simulink model "MATLAB_accumulator_tester"  (R2022a)
settings: Solver=FixedStepDiscrete  StartTime=0.0  StopTime=inf  FixedStep=Ts  MaxStep=0.001  RelTol=1e-3
PreLoadFcn:
  | load 'MATLAB_accumulator_tester_wrksp.mat'
model workspace (MAT data in the model file):
  MAX_V = Simulink.Parameter
  MAX_V.Value = 31
  MAX_V.DataType = 'single'
  MAX_V.Complexity = 'real'
  MAX_V.Dimensions = [1 1]
  MIN_ACCUM_VOLTAGE = Simulink.Parameter
  MIN_ACCUM_VOLTAGE.Value = 10
  MIN_ACCUM_VOLTAGE.DataType = 'single'
  MIN_ACCUM_VOLTAGE.Complexity = 'real'
  MIN_ACCUM_VOLTAGE.Dimensions = [1 1]
  TARGET_ACCUM_CURRENT = Simulink.Parameter
  TARGET_ACCUM_CURRENT.Value = 6
  TARGET_ACCUM_CURRENT.DataType = 'single'
  TARGET_ACCUM_CURRENT.Complexity = 'real'
  TARGET_ACCUM_CURRENT.Dimensions = [1 1]
values from neighbouring files (symbols this model uses):
  Ts = 0.01    [MATLAB_accumulator_tester_wrksp.mat]
undefined symbols (not defined in the file or in its folder): CR, d, f, LF
libraries: simulink x5, slrealtimeutilitieslib x3, instrumentlib x2, dspstat3 x2, commcrc2 x1
settings Model: SimulationMode=accelerator  Creator=DeveloperY  LastModifiedBy=DeveloperY
settings SolverCC: AllowMultiTaskInputOutput=on  ConcurrentTasks=on  AutoInsertRateTranBlk=on
settings DebuggingCC: ParameterPrecisionLossMsg=none
settings HardwareCC: ProdBitPerLong=64  ProdHWDeviceType=Intel->x86-64 (Linux 64)
settings RTWCC: Description=Simulink Desktop Real-Time  SystemTargetFile=sldrt.tlc  TemplateMakefile=sldrt.tmf  RTWCompilerOptimization=on
settings CodeAppCC: MaxIdLength=95
settings SimulinkDesktopRealTimeCC: TargetLibSuffix=_sldrt.a  TargetPreCompLibLocation=C:\Program Files\MATLAB\R2022a\toolbox\sldrt\lib\win64  RebuildAll=on

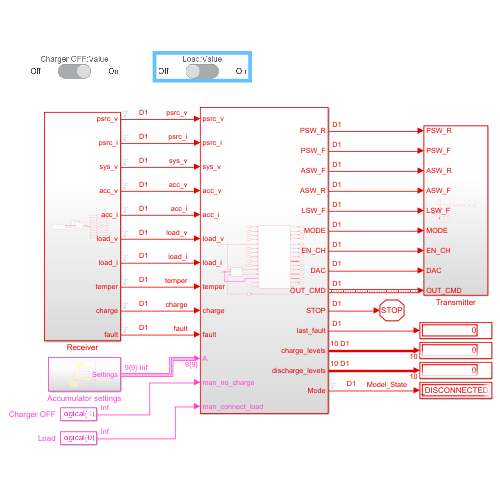
[thumbnail: Simulink's stored preview of the top-level diagram]
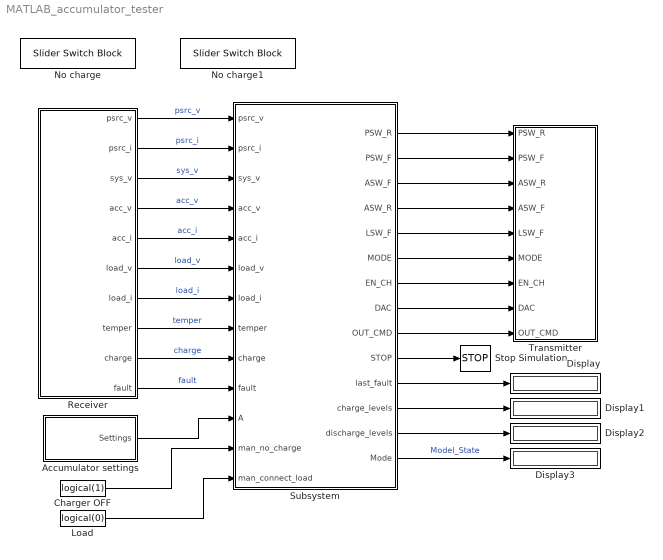
== system MATLAB_accumulator_tester ==
  Accumulator settings : Subsystem
  Charger OFF : Constant  Value=logical(1)  OutDataTypeStr=boolean
  Display{,1..3} (4 alike) : Display
  Load : Constant  Value=logical(0)  OutDataTypeStr=boolean
  No charge : SliderSwitchBlock
      settings: Values={{'Off', 'On'}, [0 1]}
  No charge1 : SliderSwitchBlock
      settings: Values={{'Off', 'On'}, [0 1]}
  Receiver : Subsystem
  Stop Simulation : Stop
  Subsystem : Subsystem
  Transmitter : Subsystem
  wires:
  Receiver/1(psrc_v) -> Subsystem/1(psrc_v)  "psrc_v"
  Receiver/2(psrc_i) -> Subsystem/2(psrc_i)  "psrc_i"
  Receiver/3(sys_v) -> Subsystem/3(sys_v)  "sys_v"
  Receiver/4(acc_v) -> Subsystem/4(acc_v)  "acc_v"
  Receiver/5(acc_i) -> Subsystem/5(acc_i)  "acc_i"
  Receiver/6(load_v) -> Subsystem/6(load_v)  "load_v"
  Receiver/7(load_i) -> Subsystem/7(load_i)  "load_i"
  Receiver/8(temper) -> Subsystem/8(temper)  "temper"
  Subsystem/1(PSW_R) -> Transmitter/1(PSW_R)
  Subsystem/2(PSW_F) -> Transmitter/2(PSW_F)
  Subsystem/3(ASW_F) -> Transmitter/3(ASW_R)
  Subsystem/4(ASW_R) -> Transmitter/4(ASW_F)
  Subsystem/5(LSW_F) -> Transmitter/5(LSW_F)
  Subsystem/6(MODE) -> Transmitter/6(MODE)
  Subsystem/7(EN_CH) -> Transmitter/7(EN_CH)
  Subsystem/8(DAC) -> Transmitter/8(DAC)
  Receiver/10(fault) -> Subsystem/10(fault)  "fault"
  Subsystem/10(" STOP") -> Stop Simulation/1
  Subsystem/11(last_fault) -> Display/1
  Accumulator settings/1(Settings) -> Subsystem/11(A)
  Receiver/9(charge) -> Subsystem/9(charge)  "charge"
  Subsystem/12(charge_levels) -> Display1/1
  Subsystem/13(discharge_levels) -> Display2/1
  Subsystem/14(Mode) -> Display3/1  "Model_State"
  Subsystem/9(OUT_CMD) -> Transmitter/9(OUT_CMD)
  Charger OFF/1 -> Subsystem/12(man_no_charge)
  Load/1 -> Subsystem/13(man_connect_load)

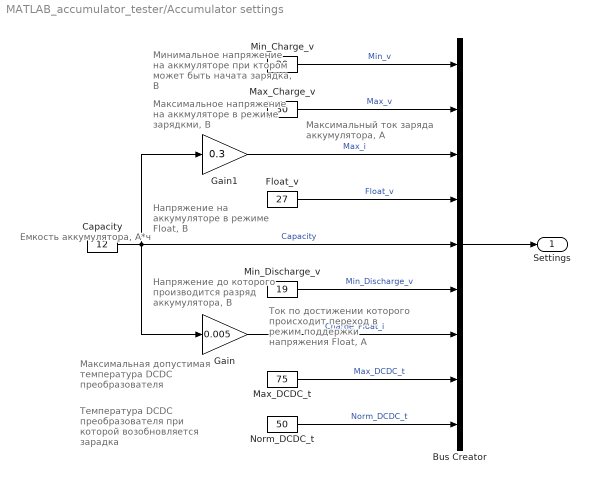
== system MATLAB_accumulator_tester/Accumulator settings ==
  note: Ток по достижении которого происходит переход в режим поддержки напряжения Float, А
  note: Максимальная допустимая температура DCDC преобразователя
  note: Температура DCDC преобразователя при которой возобновляется зарадка
  note: Напряжение до которого производится разряд аккумулятора, В
  note: Емкость аккумулятора, А*ч
  note: Напряжение на аккумуляторе в режиме Float, В
  note: Максимальное напряжение на аккмуляторе в режиме зарядкми, В
  note: Максимальный ток заряда аккумулятора, А
  note: Минимальное напряжение на аккмуляторе при ктором может быть начата зарядка, В
  Bus Creator : BusCreator  Inputs=9  OutDataTypeStr=Bus: Accum_params
  Capacity : Constant  Value=12  OutDataTypeStr=single
  Float_v : Constant  Value=27  OutDataTypeStr=single
  Gain : Gain  Gain=0.005
  Gain1 : Gain  Gain=0.3
  Max_Charge_v : Constant  Value=30  OutDataTypeStr=single
  Max_DCDC_t : Constant  Value=75  OutDataTypeStr=single
  Min_Charge_v : Constant  Value=20  OutDataTypeStr=single
  Min_Discharge_v : Constant  Value=19  OutDataTypeStr=single
  Norm_DCDC_t : Constant  Value=50  OutDataTypeStr=single
  Settings : Outport
  wires:
  Bus Creator/1 -> Settings/1
  Gain1/1 -> Bus Creator/3  "Max_i"
  Capacity/1 -> Gain/1, Gain1/1, Bus Creator/5  "Capacity"
  Max_Charge_v/1 -> Bus Creator/2  "Max_v"
  Float_v/1 -> Bus Creator/4  "Float_v"
  Min_Charge_v/1 -> Bus Creator/1  "Min_v"
  Min_Discharge_v/1 -> Bus Creator/6  "Min_Discharge_v"
  Gain/1 -> Bus Creator/7  "Charge_Float_i"
  Max_DCDC_t/1 -> Bus Creator/8  "Max_DCDC_t"
  Norm_DCDC_t/1 -> Bus Creator/9  "Norm_DCDC_t"

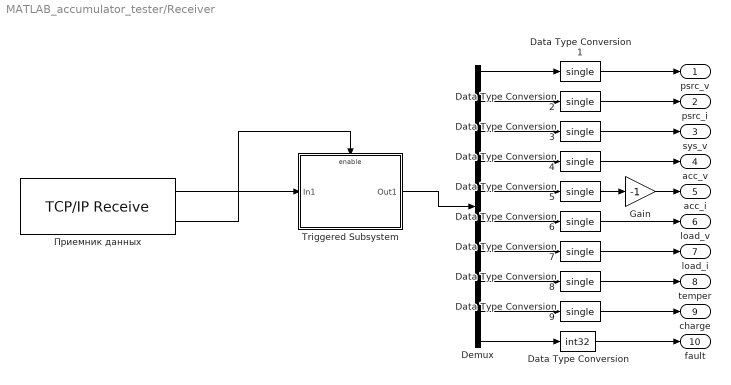
== system MATLAB_accumulator_tester/Receiver ==
  Data Type Conversion : DataTypeConversion  OutDataTypeStr=int32  SaturateOnIntegerOverflow=off  RndMeth=Floor
  Data Type Conversion{1..9} (9 alike) : DataTypeConversion  OutDataTypeStr=single  SaturateOnIntegerOverflow=off  RndMeth=Floor
  Demux : Demux  Outputs=10
  Gain : Gain  Gain=-1
  Triggered Subsystem : Subsystem  TreatAsAtomicUnit=on
  Приемник данных : instrumentlib/TCP//IP Receive  Host=192.168.3.1  Port=3333  DataSize=[10]  DataType=ASCII  ASCIIFormatting=%f,%f,%f,%f,%f,%f,%f,%f,%e,%d  Terminator=CR/LF  CustomTerminator=10  ByteOrder=big-endian  EnableBlockingMode=off  Timeout=10  SampleTime=-1  SimulateUsing=Interpreted execution
  psrc_v : Outport
  psrc_i : Outport  Port=2
  sys_v : Outport  Port=3
  acc_v : Outport  Port=4
  acc_i : Outport  Port=5
  load_v : Outport  Port=6
  load_i : Outport  Port=7
  temper : Outport  Port=8
  charge : Outport  Port=9
  fault : Outport  Port=10
  wires:
  Demux/4 -> Data Type Conversion4/1
  Demux/5 -> Data Type Conversion5/1
  Приемник данных/1 -> Triggered Subsystem/1(In1)
  Приемник данных/2 -> Triggered Subsystem/Enable
  Demux/6 -> Data Type Conversion6/1
  Demux/1 -> Data Type Conversion1/1
  Triggered Subsystem/1(Out1) -> Demux/1
  Demux/2 -> Data Type Conversion2/1
  Demux/8 -> Data Type Conversion8/1
  Demux/7 -> Data Type Conversion7/1
  Demux/3 -> Data Type Conversion3/1
  Demux/10 -> Data Type Conversion/1
  Data Type Conversion/1 -> fault/1
  Data Type Conversion1/1 -> psrc_v/1
  Data Type Conversion2/1 -> psrc_i/1
  Data Type Conversion3/1 -> sys_v/1
  Data Type Conversion4/1 -> acc_v/1
  Data Type Conversion5/1 -> Gain/1
  Data Type Conversion6/1 -> load_v/1
  Data Type Conversion7/1 -> load_i/1
  Data Type Conversion8/1 -> temper/1
  Gain/1 -> acc_i/1
  Demux/9 -> Data Type Conversion9/1
  Data Type Conversion9/1 -> charge/1

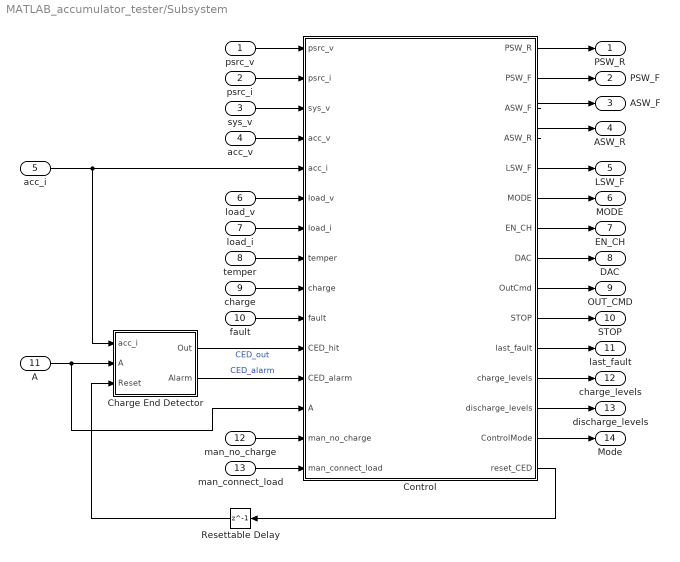
== system MATLAB_accumulator_tester/Subsystem ==
  psrc_v : Inport
  psrc_i : Inport  Port=2
  sys_v : Inport  Port=3
  acc_v : Inport  Port=4
  acc_i : Inport  Port=5
  load_v : Inport  Port=6
  load_i : Inport  Port=7
  temper : Inport  Port=8
  charge : Inport  Port=9
  fault : Inport  Port=10
  A : Inport  Port=11
  man_no_charge : Inport  Port=12
  man_connect_load : Inport  Port=13
  Charge End Detector : Subsystem
  Control : Stateflow chart  TreatAsAtomicUnit=on
  Resettable Delay : Delay  DelayLength=1
  PSW_R : Outport
  PSW_F : Outport  Port=2
  ASW_F : Outport  Port=3
  ASW_R : Outport  Port=4
  LSW_F : Outport  Port=5
  MODE : Outport  Port=6
  EN_CH : Outport  Port=7
  DAC : Outport  Port=8
  OUT_CMD : Outport  Port=9
  " STOP" : Outport  Port=10
  last_fault : Outport  Port=11
  charge_levels : Outport  Port=12
  discharge_levels : Outport  Port=13
  Mode : Outport  Port=14
  wires:
  psrc_v/1 -> Control/1(psrc_v)
  psrc_i/1 -> Control/2(psrc_i)
  sys_v/1 -> Control/3(sys_v)
  acc_v/1 -> Control/4(acc_v)
  acc_i/1 -> Charge End Detector/1(acc_i), Control/5(acc_i)
  load_v/1 -> Control/6(load_v)
  load_i/1 -> Control/7(load_i)
  temper/1 -> Control/8(temper)
  charge/1 -> Control/9(charge)
  fault/1 -> Control/10(fault)
  Charge End Detector/1(Out) -> Control/11(CED_hit)  "CED_out"
  A/1 -> Control/13(A), Charge End Detector/2(A)
  Control/1(PSW_R) -> PSW_R/1
  Control/2(PSW_F) -> PSW_F/1
  Control/3(ASW_F) -> ASW_F/1
  Control/4(ASW_R) -> ASW_R/1
  Control/5(LSW_F) -> LSW_F/1
  Control/6(MODE) -> MODE/1
  Control/7(EN_CH) -> EN_CH/1
  Control/8(DAC) -> DAC/1
  Control/10(" STOP") -> " STOP"/1
  Control/11(last_fault) -> last_fault/1
  Control/12(charge_levels) -> charge_levels/1
  Control/13(discharge_levels) -> discharge_levels/1
  Charge End Detector/2(Alarm) -> Control/12(CED_alarm)  "CED_alarm"
  Control/15(reset_CED) -> Resettable Delay/1
  Resettable Delay/1 -> Charge End Detector/3(Reset)
  Control/14(ControlMode) -> Mode/1
  Control/9(OutCmd) -> OUT_CMD/1
  man_no_charge/1 -> Control/14(man_no_charge)
  man_connect_load/1 -> Control/15(man_connect_load)

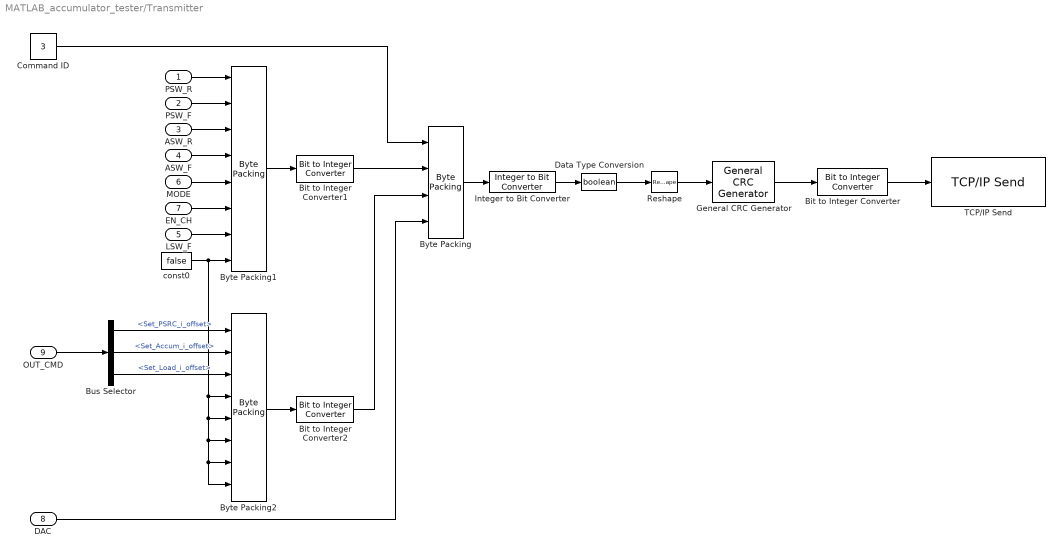
== system MATLAB_accumulator_tester/Transmitter ==
  PSW_R : Inport  OutDataTypeStr=boolean  PortDimensions=1
  PSW_F : Inport  Port=2  OutDataTypeStr=boolean  PortDimensions=1
  ASW_R : Inport  Port=3  OutDataTypeStr=boolean  PortDimensions=1
  ASW_F : Inport  Port=4  OutDataTypeStr=boolean  PortDimensions=1
  LSW_F : Inport  Port=5  OutDataTypeStr=boolean  PortDimensions=1
  MODE : Inport  Port=6  OutDataTypeStr=boolean  PortDimensions=1
  EN_CH : Inport  Port=7  OutDataTypeStr=boolean  PortDimensions=1
  DAC : Inport  Port=8  OutDataTypeStr=uint16  PortDimensions=1
  OUT_CMD : Inport  Port=9  OutDataTypeStr=Bus: OutCommands  PortDimensions=1
  Bit to Integer Converter : simulink/Logic and Bit Operations/Bit to Integer Converter  nbits=8  bitOrder=MSB first  signedOutputValues=Unsigned  outDtype=Inherit via internal rule  outDtypeSigned=Inherit via internal rule
      settings: SourceProductBaseCode=SL
  Bit to Integer Converter1 : simulink/Logic and Bit Operations/Bit to Integer Converter  nbits=8  bitOrder=LSB first  signedOutputValues=Unsigned  outDtype=Inherit via internal rule  outDtypeSigned=Inherit via internal rule
      settings: SourceProductBaseCode=SL
  Bit to Integer Converter2 : simulink/Logic and Bit Operations/Bit to Integer Converter  nbits=8  bitOrder=LSB first  signedOutputValues=Unsigned  outDtype=Inherit via internal rule  outDtypeSigned=Inherit via internal rule
      settings: SourceProductBaseCode=SL
  Bus Selector : BusSelector  OutputSignals=Set_PSRC_i_offset,Set_Accum_i_offset,Set_Load_i_offset
  Byte Packing : slrealtimeutilitieslib/Byte Packing  MaskPackedDataType=uint8  MaskUnpackedDataTypes={ 'uint32', 'uint8', 'uint8', 'uint16'}  MaskAlignment=1
  Byte Packing1 : slrealtimeutilitieslib/Byte Packing  MaskPackedDataType=boolean  MaskUnpackedDataTypes="{  'boolean', 'boolean', 'boolean', 'boolean', 'boolean', 'boolean', 'boolean', 'boolean'}"  MaskAlignment=1
  Byte Packing2 : slrealtimeutilitieslib/Byte Packing  MaskPackedDataType=boolean  MaskUnpackedDataTypes="{  'boolean', 'boolean', 'boolean', 'boolean', 'boolean', 'boolean', 'boolean', 'boolean'}"  MaskAlignment=1
  Command ID : Constant  Value=3  OutDataTypeStr=uint32
  Data Type Conversion : DataTypeConversion  OutDataTypeStr=boolean  SaturateOnIntegerOverflow=off  RndMeth=Floor
  General CRC Generator : commcrc2/General CRC Generator  genPoly='z^16 + z^12 + z^5 + 1'  iniStates=0  directMethod=off  reflectInputBytes=off  reflectChecksums=off  finalXOR=0  numChecksums=1
      settings: SourceProductBaseCode=CM
  Integer to Bit Converter : simulink/Logic and Bit Operations/Integer to Bit Converter  nbits=8  signedInputValues=Unsigned  bitOrder=MSB first  outDtype=Inherit via internal rule
      settings: SourceProductBaseCode=SL
  Reshape : Reshape  OutputDimensionality=Customize  OutputDimensions=[64,1]
  TCP/IP Send : instrumentlib/TCP//IP Send  Host=192.168.3.1  Port=3333  ByteOrder=big-endian  EnableBlockingMode=off  Timeout=0.1  TransferDelay=off  SimulateUsing=Interpreted execution
  const0 : Constant  Value=false  OutDataTypeStr=boolean
  wires:
  MODE/1 -> Byte Packing1/5
  Bit to Integer Converter1/1 -> Byte Packing/2
  Byte Packing1/1 -> Bit to Integer Converter1/1
  EN_CH/1 -> Byte Packing1/6
  PSW_F/1 -> Byte Packing1/2
  DAC/1 -> Byte Packing/4
  ASW_F/1 -> Byte Packing1/4
  PSW_R/1 -> Byte Packing1/1
  ASW_R/1 -> Byte Packing1/3
  Bit to Integer Converter/1 -> TCP/IP Send/1
  LSW_F/1 -> Byte Packing1/7
  Command ID/1 -> Byte Packing/1
  Integer to Bit Converter/1 -> Data Type Conversion/1
  General CRC Generator/1 -> Bit to Integer Converter/1
  Byte Packing/1 -> Integer to Bit Converter/1
  Reshape/1 -> General CRC Generator/1
  Data Type Conversion/1 -> Reshape/1
  OUT_CMD/1 -> Bus Selector/1
  Bus Selector/1 -> Byte Packing2/1  "<Set_PSRC_i_offset>"
  Bus Selector/2 -> Byte Packing2/2  "<Set_Accum_i_offset>"
  Bus Selector/3 -> Byte Packing2/3  "<Set_Load_i_offset>"
  const0/1 -> Byte Packing2/8, Byte Packing2/7, Byte Packing2/6, Byte Packing2/5, Byte Packing2/4, Byte Packing1/8
  Byte Packing2/1 -> Bit to Integer Converter2/1
  Bit to Integer Converter2/1 -> Byte Packing/3

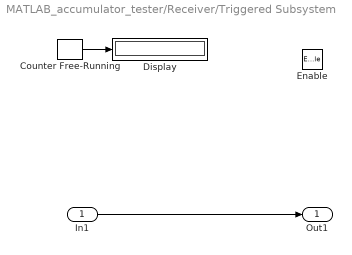
== system MATLAB_accumulator_tester/Receiver/Triggered Subsystem ==
  In1 : Inport
  Enable : EnablePort
  Counter Free-Running : simulink/Sources/Counter Free-Running  NumBits=16  tsamp=-1
  Display : Display
  Out1 : Outport
  wires:
  In1/1 -> Out1/1
  Counter Free-Running/1 -> Display/1

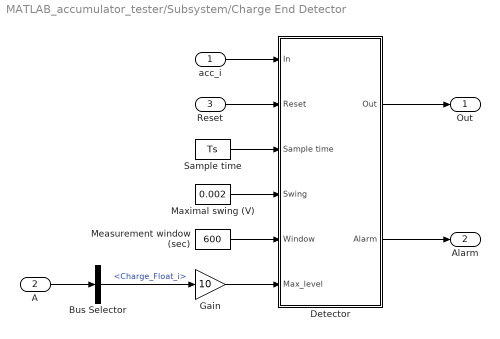
== system MATLAB_accumulator_tester/Subsystem/Charge End Detector ==
  acc_i : Inport
  A : Inport  Port=2  OutDataTypeStr=Bus: Accum_params
  Reset : Inport  Port=3
  Bus Selector : BusSelector  OutputSignals=Charge_Float_i
  Detector : Subsystem
  Gain : Gain  Gain=10
  Maximal swing (V) : Constant  Value=0.002  OutDataTypeStr=single
  Measurement window (sec) : Constant  Value=600  OutDataTypeStr=single
  Sample time : Constant  Value=Ts  OutDataTypeStr=single
  Out : Outport  OutDataTypeStr=boolean
  Alarm : Outport  Port=2  OutDataTypeStr=boolean
  wires:
  Measurement window (sec)/1 -> Detector/5(Window)
  Sample time/1 -> Detector/3(Sample time)
  Maximal swing (V)/1 -> Detector/4(Swing)
  acc_i/1 -> Detector/1(In)
  Reset/1 -> Detector/2(Reset)
  Detector/1(Out) -> Out/1
  Detector/2(Alarm) -> Alarm/1
  A/1 -> Bus Selector/1
  Bus Selector/1 -> Gain/1  "<Charge_Float_i>"
  Gain/1 -> Detector/6(Max_level)

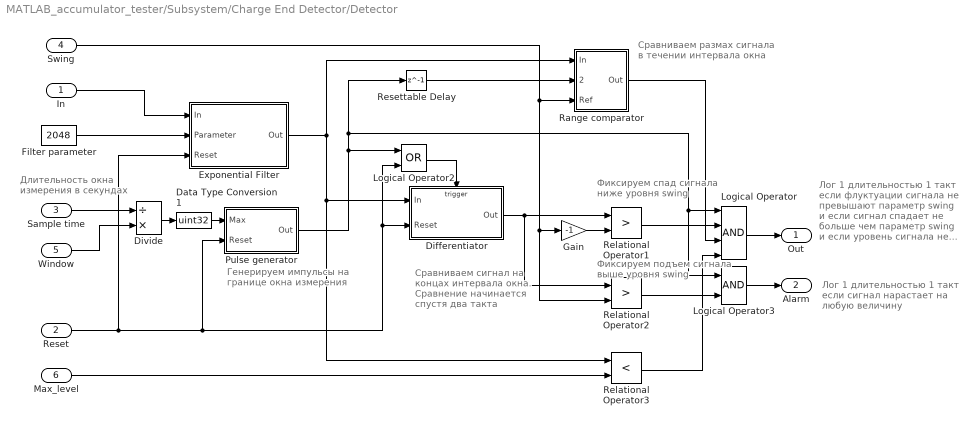
== system MATLAB_accumulator_tester/Subsystem/Charge End Detector/Detector ==
  note: Длительность окна измерения в секундах
  note: Сравниваем сигнал на концах интервала окна.
      | Сравнение начинается спустя два такта
  note: Сравниваем размах сигнала в течении интервала окна
  note: Лог 1 длительностью 1 такт если сигнал нарастает на любую величину
  note: Фиксируем спад сигнала ниже уровня swing
  note: Лог 1 длительностью 1 такт если флуктуации сигнала не превышают параметр swing
      | и если сигнал спадает не больше чем параметр swing и если уровень сигнала не превышает Max_level
  note: Генерируем импульсы на границе окна измерения
  note: Фиксируем подъем сигнала выше уровня swing
  In : Inport  OutDataTypeStr=single  SampleTime=0.01
  Reset : Inport  Port=2  OutDataTypeStr=boolean  SampleTime=0.01
  Sample time : Inport  Port=3  OutDataTypeStr=single  SampleTime=0.01
  Swing : Inport  Port=4  OutDataTypeStr=single  SampleTime=0.01
  Window : Inport  Port=5  OutDataTypeStr=single  SampleTime=0.01
  Max_level : Inport  Port=6  OutDataTypeStr=single  SampleTime=0.01
  Data Type Conversion1 : DataTypeConversion  OutDataTypeStr=uint32  SaturateOnIntegerOverflow=off  RndMeth=Floor
  Differentiator : Subsystem  TreatAsAtomicUnit=on
  Divide : Product  Inputs=/*
  Exponential Filter : Subsystem
  Filter parameter : Constant  Value=2048  OutDataTypeStr=single
  Gain : Gain  Gain=-1
  Logical Operator : Logic  Inputs=4  AllPortsSameDT=off  OutDataTypeStr=boolean
  Logical Operator2 : Logic  Operator=OR  AllPortsSameDT=off  OutDataTypeStr=boolean
  Logical Operator3 : Logic  AllPortsSameDT=off  OutDataTypeStr=boolean
  Pulse generator : Subsystem
  Range comparator : Subsystem
  Relational Operator1 : RelationalOperator  Operator=>  OutDataTypeStr=boolean  RndMeth=Simplest
  Relational Operator2 : RelationalOperator  Operator=>  OutDataTypeStr=boolean  RndMeth=Simplest
  Relational Operator3 : RelationalOperator  Operator=<  OutDataTypeStr=boolean  RndMeth=Simplest
  Resettable Delay : Delay  DelayLength=1
  Out : Outport
  Alarm : Outport  Port=2
  wires:
  Sample time/1 -> Divide/1
  Divide/1 -> Data Type Conversion1/1
  Pulse generator/1(Out) -> Resettable Delay/1, Logical Operator3/1, Logical Operator/1, Logical Operator2/1
  Window/1 -> Divide/2
  In/1 -> Exponential Filter/1(In)
  Data Type Conversion1/1 -> Pulse generator/1(Max)
  Exponential Filter/1(Out) -> Range comparator/1(In), Relational Operator3/1, Differentiator/1(In)
  Relational Operator1/1 -> Logical Operator/2
  Range comparator/1(Out) -> Logical Operator/3
  Logical Operator/1 -> Out/1
  Reset/1 -> Logical Operator2/2, Differentiator/2(Reset), Pulse generator/2(Reset), Exponential Filter/3(Reset)
  Filter parameter/1 -> Exponential Filter/2(Parameter)
  Differentiator/1(Out) -> Relational Operator1/1, Relational Operator2/1
  Resettable Delay/1 -> Range comparator/2(Reset)
  Relational Operator2/1 -> Logical Operator3/2
  Logical Operator2/1 -> Differentiator/Trigger
  Logical Operator3/1 -> Alarm/1
  Swing/1 -> Range comparator/3(Ref), Gain/1, Relational Operator2/2
  Gain/1 -> Relational Operator1/2
  Max_level/1 -> Relational Operator3/2
  Relational Operator3/1 -> Logical Operator/4

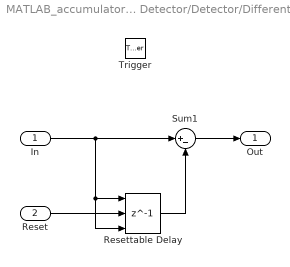
== system MATLAB_accumulator_tester/Subsystem/Charge End Detector/Detector/Differentiator ==
  In : Inport
  Reset : Inport  Port=2
  Trigger : TriggerPort  VariantControl=(inherit)
  Resettable Delay : Delay  DelayLength=1  InitialConditionSource=Input port  ExternalReset=Level
      settings: InputPortMap=u0,r5,p4
  Sum1 : Sum  Inputs=|+-
  Out : Outport  SourceOfInitialOutputValue=Input signal
  wires:
  In/1 -> Resettable Delay/3, Resettable Delay/1, Sum1/1
  Resettable Delay/1 -> Sum1/2
  Sum1/1 -> Out/1
  Reset/1 -> Resettable Delay/2

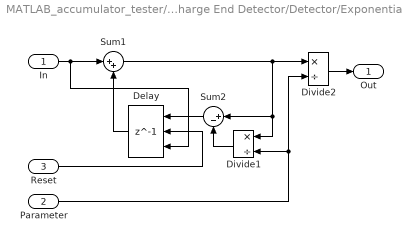
== system MATLAB_accumulator_tester/Subsystem/Charge End Detector/Detector/Exponential Filter ==
  In : Inport
  Parameter : Inport  Port=2
  Reset : Inport  Port=3
  Delay : Delay  DelayLength=1  InitialConditionSource=Input port  InitialCondition=0  ExternalReset=Rising
      settings: InputPortMap=u0,r5,p4
  Divide1 : Product  Inputs=*/
  Divide2 : Product  Inputs=*/
  Sum1 : Sum  Inputs=|++
  Sum2 : Sum  Inputs=|+-
  Out : Outport
  wires:
  Divide2/1 -> Out/1
  Divide1/1 -> Sum2/2
  Parameter/1 -> Divide1/2, Divide2/2
  In/1 -> Delay/3, Sum1/1
  Sum2/1 -> Delay/1
  Delay/1 -> Sum1/2
  Sum1/1 -> Divide2/1, Divide1/1, Sum2/1
  Reset/1 -> Delay/2

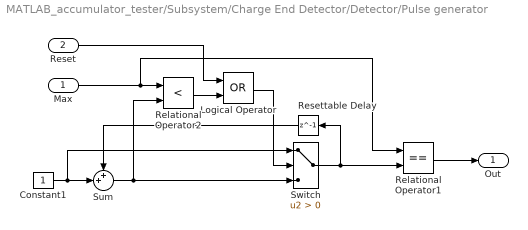
== system MATLAB_accumulator_tester/Subsystem/Charge End Detector/Detector/Pulse generator ==
  Max : Inport
  Reset : Inport  Port=2
  Constant1 : Constant  OutDataTypeStr=uint32
  Logical Operator : Logic  Operator=OR  AllPortsSameDT=off  OutDataTypeStr=boolean
  Relational Operator1 : RelationalOperator  Operator===  OutDataTypeStr=boolean  RndMeth=Simplest
  Relational Operator2 : RelationalOperator  Operator=<  OutDataTypeStr=boolean  RndMeth=Simplest
  Resettable Delay : Delay  DelayLength=1
  Sum : Sum  Inputs=++|
  Switch : Switch  Criteria=u2 > Threshold  SaturateOnIntegerOverflow=off  InputSameDT=off
  Out : Outport
  wires:
  Sum/1 -> Switch/3, Relational Operator2/2
  Max/1 -> Relational Operator1/1, Relational Operator2/1
  Switch/1 -> Resettable Delay/1, Relational Operator1/2
  Resettable Delay/1 -> Sum/1
  Constant1/1 -> Sum/2, Switch/1
  Relational Operator2/1 -> Logical Operator/2
  Reset/1 -> Logical Operator/1
  Logical Operator/1 -> Switch/2
  Relational Operator1/1 -> Out/1

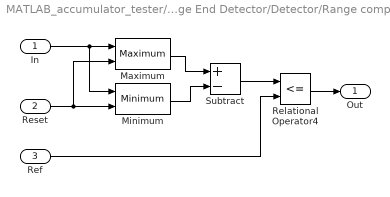
== system MATLAB_accumulator_tester/Subsystem/Charge End Detector/Detector/Range comparator ==
  In : Inport
  Reset : Inport  Port=2
  Ref : Inport  Port=3
  Maximum : dspstat3/Maximum  operation=maximum  fcn=Running  indexBase=One  operateOver=Each column  Dimension=1  reset=Rising edge  roiEnable=off  roiType=Rectangles  roiPortion=Entire ROI  roiOutput=Individual statistics for each ROI  roiFlag=off  roundingMode=Floor  overflowMode=off  accumDataTypeStr=Inherit: Same as product output  accumLastDataTypeStr=Inherit: Same as product output
  Minimum : dspstat3/Minimum  operation=minimum  fcn=Running  indexBase=One  operateOver=Each column  Dimension=1  reset=Rising edge  roiEnable=off  roiType=Rectangles  roiPortion=Entire ROI  roiOutput=Individual statistics for each ROI  roiFlag=off  roundingMode=Floor  overflowMode=off
      settings: SourceProductBaseCode=DS
  Relational Operator4 : RelationalOperator  Operator=<=  OutDataTypeStr=boolean  RndMeth=Simplest
  Subtract : Sum  Inputs=+-
  Out : Outport
  wires:
  Reset/1 -> Maximum/2, Minimum/2
  In/1 -> Minimum/1, Maximum/1
  Maximum/1 -> Subtract/1
  Minimum/1 -> Subtract/2
  Subtract/1 -> Relational Operator4/1
  Relational Operator4/1 -> Out/1
  Ref/1 -> Relational Operator4/2

== stateflow chart MATLAB_accumulator_tester/Subsystem/Control ==
  settings: sampleTime=0.01
  state Continues_mode [function]
    (default) -> (junction 236) : {MODE = false;}
  state PREPARATION
    state S0
      state S1
        en:
        PSW_R = true;
        PSW_F = true;
        ASW_F = false;
        ASW_R = false;
        LSW_F = false;
        PulseSkiping_mode;
        EN_CH = false;
        DAC = V_to_DAC(single(0));
      state S2
        en:
        OutCmd.Set_Load_i_offset=true;
        OutCmd.Set_Accum_i_offset=true;
      state S3
        en:
        OutCmd.Set_Load_i_offset=false;
        OutCmd.Set_Accum_i_offset=false;
        PSW_R = false;
      state S4
        en:
        ASW_F = true;
      state S5
        en:
        PSW_F = false;
        ASW_R = true;
      state S6
        en:
        OutCmd.Set_PSRC_i_offset=true;
      state S7
        en:
        OutCmd.Set_PSRC_i_offset=false;
        ASW_R = false;
      state S8
        en:
        PSW_F = true;
      state S9
        en:
        ASW_F = false;
      state S10
        en:
        PSW_R = true;
      S1 -> S2 : after(0.3,sec)
      S2 -> S3
      S3 -> S4
      S4 -> S5
      S5 -> S6 : after(0.3,sec)
      S6 -> S7
      S7 -> S8
      S8 -> S9
      S9 -> S10
    note: Источник питания подключаем. Нагрузку и аккумулятор отклюсчаем
    note: Выдаем команду на корректировку смещений нуля измерителям тока аккумулятора и нагрузки
    note: Оставляем источник питания подключенный к системной шине через диод
    note: Подключаем акумулятор к системной шине через диод
    note: Полностью отключаем источник питания, и полностью подключаем аккумулятор к системной шине
    note: Выдаем команду на корректировку смещений нуля измерителям тока источника питания
    note: Оставляем акумулятор подключенным к системной шине через диод
    note: Подключаем источник питания к системной шине через диод
    note: Полностью отключаем аккумулятор
    note: Полностью включаем источник питания
    (default) -> S1
    S0 -> 366 : [(acc_v < A.Min_v) ||  (psrc_v < 20.0) ]
    S10 -> 369
  state PulseSkiping_mode [function]
    (default) -> (junction 239) : {MODE = true;}
  note: Самодиагностика, калибровка и настройка
  state MAIN
    state AUTO
      state CHARGING
        en:
        init_charge = charge;
        delta_charge=0;
        du: delta_charge=charge-init_charge;
        state PSRC_PREPARING
          en:
          PSW_R = true;
          PSW_F = true;
          PulseSkiping_mode;
          EN_CH = false;
          note: Подключаем источник питания
        state DCDC_Mode_control [function]
          (default) -> (junction 251) : [MODE==true]
          (junction 251) -> (junction 256) : [acc_i>1.0]
          (junction 256) -> (junction 253) : {Continues_mode;}
        state CHARGE_PROCESS
          state SET_INIT_VOLTAGE
            en:
            reset_CED = true;
            PulseSkiping_mode;
            voltage_setting = acc_v - single(0.2);
            DAC = V_to_DAC(voltage_setting);
            note: Подготовка к включению зарядника.
          state FAST_CHARGING
            state CONST_CURRENT
              du:
              Set_current(A.Max_i, 0.001);
              note: Зарядка константным током, напряжение растет
            state CONST_VOLTAGE
              en: reset_CED = false;
              note: Зарядка константным напряжением, ток спадает.
                  | Здесь следим за скоростью спада тока
            CONST_CURRENT -> CONST_VOLTAGE : [acc_i < (A.Max_i*0.9)]
          state SET_INIT_CURRENT
            en:
            EN_CH = true;
            du:
            Set_current( A.Charge_Float_i, 0.01);
            note: Устанавливаем начальный ток грубо
          note: Аккумулятор либо не подключен либо имеет слишком высокое сопротивление
          state SET_TARGET_CURRENT
            du:
            Set_current(A.Max_i, 0.001);
            DCDC_Mode_control;
            note: Поднимаем напряжение до максимума, пока не установится максимальный ток
          state RELAX
            en:
            EN_CH = false; reset_CED = true;
            PulseSkiping_mode;
            voltage_setting = A.Float_v;
            DAC = V_to_DAC(voltage_setting);
            note: Отключаем зарядку, ждём пока напряжение упадет до уровня Float_v
          state FLOAT
            en:
            EN_CH = true; reset_CED = false;
            du:
            DCDC_Mode_control;
            note: Включаем зарядку на уровень поддержки напряжения = Float_v
          SET_INIT_VOLTAGE -> SET_INIT_CURRENT : after(0.05, sec)
          (junction 336) -> CONST_CURRENT
          (junction 333) -> (junction 336)
          SET_INIT_CURRENT -> (junction 160) [order 2] : [acc_v >= A.Max_v]
          (junction 160) -> RELAX
          SET_INIT_CURRENT -> SET_TARGET_CURRENT [order 1] : [duration(acc_i >= A.Charge_Float_i, sec)>60]
          SET_TARGET_CURRENT -> (junction 333) [order 1] : [acc_i >= A.Max_i]
          SET_TARGET_CURRENT -> CONST_VOLTAGE [order 2] : [voltage_setting >= A.Max_v]
          CONST_VOLTAGE -> (junction 321)
          FAST_CHARGING -> (junction 327)
          (junction 327) -> RELAX [order 1] : [acc_i < A.Charge_Float_i]
          (junction 327) -> (junction 328) [order 2]
          (junction 328) -> RELAX [order 1] : [delta_charge>(A.Capacity*1.1)]
          (junction 328) -> (junction 329) [order 2]
          (junction 329) -> RELAX : [CED_hit]
          RELAX -> FLOAT : [acc_v < (voltage_setting-0.1)]
          FLOAT -> (junction 321) [order 3]
        state COOLING_WAITING
          en:
          EN_CH = false;
          PulseSkiping_mode;
          note: Пауза процесса зарядки для защиты от перегрева DCDC преобразователя
        state CHARGE_END
          en:
          EN_CH = false;
          PulseSkiping_mode;
          note: Выключаем зарядку спустя некоторое время
        (default) -> PSRC_PREPARING
        PSRC_PREPARING -> SET_INIT_VOLTAGE : after(0.1, sec)
        COOLING_WAITING -> SET_INIT_VOLTAGE : [temper < A.Norm_DCDC_t]
        (junction 340) -> COOLING_WAITING
        CHARGE_PROCESS -> (junction 340) : [temper > A.Max_DCDC_t]
        (junction 321) -> (junction 319) : [CED_alarm]
        FLOAT -> CHARGE_END [order 2] : [delta_charge>(A.Capacity*1.1)]
        FLOAT -> CHARGE_END [order 1] : after(1800, sec)
        (junction 319) -> CHARGE_END
        CHARGE_END -> (junction 293) : after(60, sec)
        (junction 293) -> 272 : {charge_levels(cycle_counter) = delta_charge;}
      state DISCHARGE
        en:
        EN_CH = false;
        PulseSkiping_mode;
        init_charge = charge;  delta_charge=0;
        du:
        delta_charge=charge-init_charge;
        note: Включаем разряд аккумулятора
        state DISCHARGE
          en:
          LSW_F=true;
        state DISCONNECTED
          en:
          LSW_F=false;
        (default) -> MAIN.AUTO.DISCHARGE.DISCHARGE
        MAIN.AUTO.DISCHARGE.DISCHARGE -> DISCONNECTED : [acc_v < A.Min_Discharge_v]
        DISCONNECTED -> (junction 295) : after(60,sec)
        (junction 295) -> 259 : {discharge_levels(cycle_counter) = delta_charge;}
      (default) -> CHARGING
      104 -> MAIN.AUTO.DISCHARGE
    state MANUAL
      en:
      EN_CH = false;
      LSW_F=false;
      PulseSkiping_mode;
      du:
      delta_charge=charge-init_charge;
      state MAN
        state LOAD_MAN_DISCONNECTED
          en:
          LSW_F=false;
        state LOAD_MAN_CONNECTED
          en:
          LSW_F=true;
        (default) -> LOAD_MAN_DISCONNECTED
        LOAD_MAN_DISCONNECTED -> LOAD_MAN_CONNECTED : [man_connect_load]
        LOAD_MAN_CONNECTED -> LOAD_MAN_DISCONNECTED : [~man_connect_load]
      state MAN_EXIT
      (default) -> MAN
      MAN -> (junction 421) : [~man_no_charge]
      (junction 421) -> MAN_EXIT : {LSW_F=false;}
      MAN_EXIT -> 417 : after(0.1,sec)
    (default) -> AUTO
    (junction 269) -> CHARGING
    (junction 267) -> (junction 269)
    AUTO -> MANUAL : [man_no_charge]
    418 -> AUTO
    263 -> (junction 265) : {cycle_counter = cycle_counter + 1;}
    (junction 265) -> (junction 267) [order 2]
  note: Слишком низкое напряжение источника питания
  note: Внутренняя ошибка DCDC конвертера
  note: Обнаружен втекающий ток аккумулятора
  note: Слишком низкое напряжение аккумулятора
  state STOP
    en:
    PSW_R = false;
    PSW_F = false;
    ASW_F = false;
    ASW_R = false;
    LSW_F = false;
    MODE = true;
    EN_CH = false;
    DAC = V_to_DAC(single(0));
  (default) -> PREPARATION
  367 -> (junction 373) : {last_fault=103}
  (junction 373) -> (junction 89)
  370 -> MAIN : {cycle_counter=1;}
  MAIN -> (junction 89) [order 1] : [ psrc_v < single(20) ]{last_fault=100}
  (junction 89) -> (junction 91)
  MAIN -> (junction 91) [order 3] : [fault~=0]{last_fault=fault}
  (junction 91) -> (junction 168)
  MAIN -> (junction 168) [order 4] : [-acc_i>0.2]{last_fault=101}
  (junction 168) -> (junction 227)
  MAIN -> (junction 227) [order 2] : [acc_v < A.Min_v]{last_fault=102}
  (junction 227) -> STOP
  (junction 265) -> STOP [order 1] : [cycle_counter>10]{last_fault=0}
  data: voltage function_input; val function_output; current function_input; step function_input; PSW_R output boolean =false; PSW_F output boolean =false; ASW_F output boolean =false; ASW_R output boolean =false; LSW_F output boolean =false; MODE output boolean =false; EN_CH output boolean =false; DAC output uint16 =uint16(0xFFFF); OutCmd output Bus: OutCommands; psrc_v input single; psrc_i input single; sys_v input single; acc_v input single; acc_i input single; load_v input single; load_i input single; temper input single; charge input single; fault input int32; CED_hit input boolean; STOP output boolean; voltage_setting local single =single(0); last_fault output int32 size=1; init_charge local single =single(0); delta_charge local single =single(0); cycle_counter local int32 =int32(0); charge_levels output single size=10; discharge_levels output single size=10; ControlMode output Enum: ControlModeType; reset_CED output boolean =false; CED_alarm input boolean; A input Bus: Accum_params; man_no_charge input boolean; man_connect_load input boolean
  function val = V_to_DAC(voltage):
    | function val = V_to_DAC(voltage)
    | 
    | 
    | MIN_VOUT = single(1.3);
    | MAX_VOUT = single(32.51);
    | SWING_V  = single(MAX_VOUT - MIN_VOUT);
    | 
    | if voltage < MIN_VOUT
    |     voltage = MIN_VOUT;
    | end
    | 
    | if voltage > MAX_VOUT
    |     voltage = MAX_VOUT;
    | end
    | 
    | 
    | val = uint16(uint16(0xFFFF) - uint16(  (single(voltage)-MIN_VOUT) * single(65535) / SWING_V ) );
    | 
    | end
  function Set_current(current, step):
    | function Set_current(current, step)
    |  
    | if acc_i < current
    |     if voltage_setting < A.Max_v
    |         voltage_setting=voltage_setting+step;
    |     end
    |     DAC = V_to_DAC(voltage_setting);
    | end
